simulink model "osc"  (Simulink 2.09)
settings: Solver=FixedStepDiscrete  StartTime=0.0  StopTime=999999  RelTol=1e-3  AbsTol=1e-6
undefined symbols (not defined in the file): rad, sec
libraries: dspsnks x1, dspspect x1, dspelmat x1
settings Model: SaveTime=off  SaveOutput=off  ConsistencyChecking=off  RTWTemplateMakefile=grt_vc.tmf

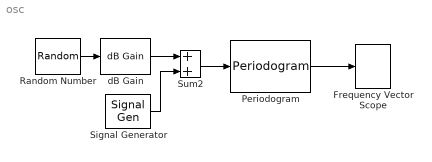
== system osc ==
  Frequency Vector Scope : dspsnks/Frequency Vector Scope  radsPop=rad/sec  frange=Half  ampl_scale=dB  ylabel=Magnitude, dB  figpos=[50 100 400 250]  ts=1
  Periodogram : dspspect/Periodogram  bufsiz=128  olap=64  fftsize=128  navg=4  wintype=Hamming  Rs=50  beta=5  winsamp=Symmetric  Ts=1
  Random Number : RandomNumber  Mean=0  Variance=1  Seed=0  SampleTime=1
  Signal Generator : SignalGenerator  WaveForm=sine  Amplitude=1.000000  Frequency=1.5  Units=rad/sec
  Sum2 : Sum  Inputs=++
  dB Gain : dspelmat/dB Gain  dB=-20  intype=Amplitude
  wires:
  Periodogram/1 -> Frequency Vector Scope/1
  dB Gain/1 -> Sum2/1
  Random Number/1 -> dB Gain/1
  Sum2/1 -> Periodogram/1
  Signal Generator/1 -> Sum2/2
